simulink model "tf6MayAgain"  (R2017b)
settings: Solver=VariableStepAuto  StartTime=0.0  StopTime=40  MaxStep=1e-4  RelTol=1e-3
libraries: powerlib x1
settings Model: Creator=bikulborthakur  LastModifiedBy=bikulborthakur

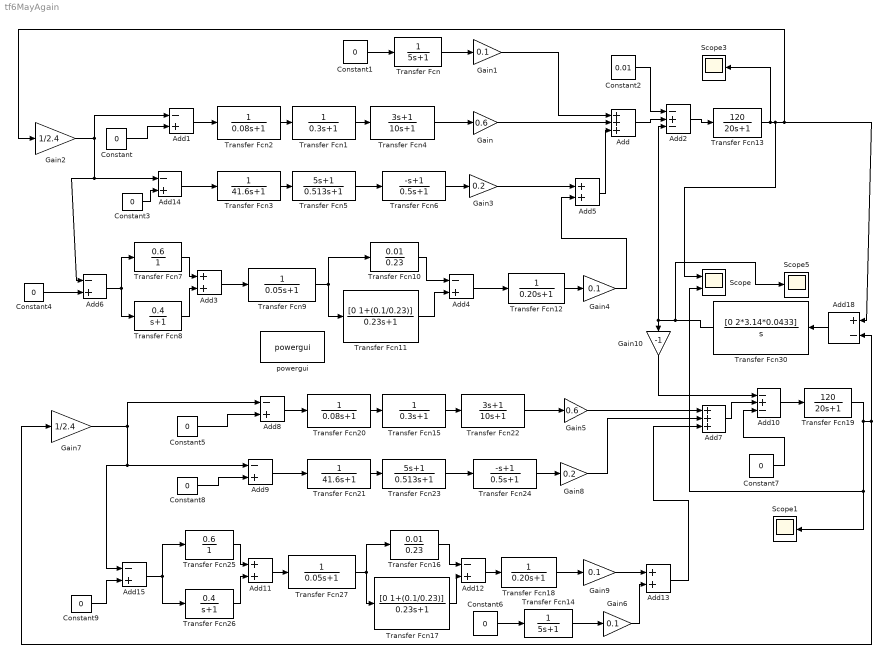
== system tf6MayAgain ==
  Add : Sum  Inputs=+++
  Add{1,4,6,8..9,12,14..15} (8 alike) : Sum  Inputs=-+
  Add10 : Sum  Inputs=-+-
  Add{3,5,11,13} (4 alike) : Sum
  Add18 : Sum  Inputs=+-
  Add2 : Sum  Inputs=-+-
  Add7 : Sum  Inputs=+++
  Constant{,1,3..9} (9 alike) : Constant  Value=0
  Constant2 : Constant  Value=0.01
  Gain : Gain  Gain=0.6
  Gain{1,4,6,9} (4 alike) : Gain  Gain=0.1
  Gain10 : Gain  Gain=-1
  Gain2 : Gain  Gain=1/2.4
  Gain3 : Gain  Gain=0.2
  Gain5 : Gain  Gain=0.6
  Gain7 : Gain  Gain=1/2.4
  Gain8 : Gain  Gain=0.2
  Scope : Scope  NumInputPorts=2
  Scope1 : Scope
  Scope3 : Scope
  Scope5 : Scope
  Transfer Fcn : TransferFcn  Denominator=[5 1]
  Transfer Fcn1 : TransferFcn  Numerator=[0 1]  Denominator=[0.3 1]
  Transfer Fcn10 : TransferFcn  Numerator=[0 0.01]  Denominator=[0 0.23]
  Transfer Fcn11 : TransferFcn  Numerator=[0 1+(0.1/0.23)]  Denominator=[0.23 1]
  Transfer Fcn12 : TransferFcn  Denominator=[0.20 1]
  Transfer Fcn13 : TransferFcn  Numerator=[0 120]  Denominator=[20 1]
  Transfer Fcn14 : TransferFcn  Denominator=[5 1]
  Transfer Fcn15 : TransferFcn  Numerator=[0 1]  Denominator=[0.3 1]
  Transfer Fcn16 : TransferFcn  Numerator=[0 0.01]  Denominator=[0 0.23]
  Transfer Fcn17 : TransferFcn  Numerator=[0 1+(0.1/0.23)]  Denominator=[0.23 1]
  Transfer Fcn18 : TransferFcn  Denominator=[0.20 1]
  Transfer Fcn19 : TransferFcn  Numerator=[0 120]  Denominator=[20 1]
  Transfer Fcn2 : TransferFcn  Numerator=[0 1]  Denominator=[0.08 1]
  Transfer Fcn20 : TransferFcn  Numerator=[0 1]  Denominator=[0.08 1]
  Transfer Fcn21 : TransferFcn  Denominator=[41.6 1]
  Transfer Fcn22 : TransferFcn  Numerator=[3 1]  Denominator=[10 1]
  Transfer Fcn23 : TransferFcn  Numerator=[5 1]  Denominator=[0.513 1]
  Transfer Fcn24 : TransferFcn  Numerator=[-1 1]  Denominator=[0.5 1]
  Transfer Fcn25 : TransferFcn  Numerator=[0 0.6]  Denominator=[0 1]
  Transfer Fcn26 : TransferFcn  Numerator=[0 0.4]  Denominator=[1 1]
  Transfer Fcn27 : TransferFcn  Denominator=[0.05 1]
  Transfer Fcn3 : TransferFcn  Denominator=[41.6 1]
  Transfer Fcn30 : TransferFcn  Numerator=[0 2*3.14*0.0433]  Denominator=[1 0]
  Transfer Fcn4 : TransferFcn  Numerator=[3 1]  Denominator=[10 1]
  Transfer Fcn5 : TransferFcn  Numerator=[5 1]  Denominator=[0.513 1]
  Transfer Fcn6 : TransferFcn  Numerator=[-1 1]  Denominator=[0.5 1]
  Transfer Fcn7 : TransferFcn  Numerator=[0 0.6]  Denominator=[0 1]
  Transfer Fcn8 : TransferFcn  Numerator=[0 0.4]  Denominator=[1 1]
  Transfer Fcn9 : TransferFcn  Denominator=[0.05 1]
  powergui : powerlib/powergui  Priority=1  SimulationMode=Continuous  SampleTime=0.001  frequency=60  Iterations=50  frequencyindice=60  Pbase=100e6  ErrMax=1e-4  UnitsV=kV  UnitsW=MW  buscounter=0  FunctionMessages=off  echomessages=off  EnableUseOfTLC=off  CurrentSourceSwitches=off  DisableSnubberDevices=off  DisableRonSwitches=off  DisableVfSwitches=off  DisplayEquations=off  SolverType=Tustin/Backward Euler (TBE)  Interpol=off  ExternalGateDelay=off  methode=off  Ts=100  x0status=blocks  SPID=on  SwTol=0  HookPort=off  RestoreLinks=warning  ResistiveCurrentMeasurement=off  Frange=[0:2:500]  Ylog=off  Xlog=on  ShowGrid=off  save=off  variable=ZData  structure=0  ZoomFFT=off  StartTime=0.0  cycles=1  DisplayStyle=1  fundamental=60  FreqAxis=off  MaxFrequency=1000  frequencyindicesteady=1  RmsSteady=1  display=off
  wires:
  Transfer Fcn13/1 -> Add18/1, Gain2/1, Scope/1, Scope3/1
  Constant9/1 -> Add15/2
  Add5/1 -> Add/3
  Add6/1 -> Transfer Fcn8/1, Transfer Fcn7/1
  Transfer Fcn16/1 -> Add12/1
  Gain5/1 -> Add7/1
  Constant1/1 -> Transfer Fcn/1
  Transfer Fcn3/1 -> Transfer Fcn5/1
  Constant8/1 -> Add9/2
  Add4/1 -> Transfer Fcn12/1
  Add1/1 -> Transfer Fcn2/1
  Transfer Fcn18/1 -> Gain9/1
  Transfer Fcn22/1 -> Gain5/1
  Transfer Fcn11/1 -> Add4/2
  Transfer Fcn1/1 -> Transfer Fcn4/1
  Constant5/1 -> Add8/2
  Transfer Fcn10/1 -> Add4/1
  Add14/1 -> Transfer Fcn3/1
  Add18/1 -> Transfer Fcn30/1
  Transfer Fcn8/1 -> Add3/2
  Gain2/1 -> Add6/1, Add14/1, Add1/1
  Transfer Fcn12/1 -> Gain4/1
  Add13/1 -> Add7/3
  Gain7/1 -> Add8/1, Add9/1, Add15/1
  Gain9/1 -> Add13/1
  Transfer Fcn25/1 -> Add11/1
  Transfer Fcn26/1 -> Add11/2
  Add15/1 -> Transfer Fcn26/1, Transfer Fcn25/1
  Gain6/1 -> Add13/2
  Add9/1 -> Transfer Fcn21/1
  Constant7/1 -> Add10/3
  Transfer Fcn5/1 -> Transfer Fcn6/1
  Transfer Fcn4/1 -> Gain/1
  Constant/1 -> Add1/2
  Transfer Fcn24/1 -> Gain8/1
  Transfer Fcn27/1 -> Transfer Fcn17/1, Transfer Fcn16/1
  Add10/1 -> Transfer Fcn19/1
  Transfer Fcn6/1 -> Gain3/1
  Transfer Fcn19/1 -> Scope1/1, Scope/2, Add18/2, Gain7/1
  Add8/1 -> Transfer Fcn20/1
  Transfer Fcn/1 -> Gain1/1
  Constant3/1 -> Add14/2
  Transfer Fcn17/1 -> Add12/2
  Gain1/1 -> Add/1
  Add12/1 -> Transfer Fcn18/1
  Constant2/1 -> Add2/1
  Gain8/1 -> Add7/2
  Constant6/1 -> Transfer Fcn14/1
  Add2/1 -> Transfer Fcn13/1
  Transfer Fcn2/1 -> Transfer Fcn1/1
  Gain3/1 -> Add5/1
  Transfer Fcn20/1 -> Transfer Fcn15/1
  Add/1 -> Add2/2
  Add3/1 -> Transfer Fcn9/1
  Transfer Fcn9/1 -> Transfer Fcn11/1, Transfer Fcn10/1
  Add11/1 -> Transfer Fcn27/1
  Add7/1 -> Add10/2
  Constant4/1 -> Add6/2
  Transfer Fcn23/1 -> Transfer Fcn24/1
  Transfer Fcn14/1 -> Gain6/1
  Gain4/1 -> Add5/2
  Transfer Fcn15/1 -> Transfer Fcn22/1
  Gain/1 -> Add/2
  Transfer Fcn21/1 -> Transfer Fcn23/1
  Transfer Fcn7/1 -> Add3/1
  Gain10/1 -> Add10/1
  Transfer Fcn30/1 -> Scope5/1, Add2/3, Gain10/1
